simulink model "lab03part1"  (R2015a)
settings: Solver=ode45  StartTime=0.0  StopTime=40.0  RelTol=1e-3
settings Model: Creator=dg  LastModifiedBy=dg

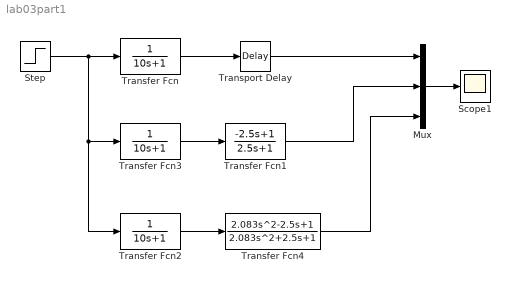
== system lab03part1 ==
  Mux : Mux  Inputs=3
  Scope1 : Scope
  Step : Step  SampleTime=0
  Transfer Fcn : TransferFcn  Denominator=[10 1]
  Transfer Fcn1 : TransferFcn  Numerator=[-2.5 1]  Denominator=[2.5 1]
  Transfer Fcn2 : TransferFcn  Denominator=[10 1]
  Transfer Fcn3 : TransferFcn  Denominator=[10 1]
  Transfer Fcn4 : TransferFcn  Numerator=[2.083 -2.5 1]  Denominator=[2.083 2.5 1]
  Transport Delay : TransportDelay
  wires:
  Step/1 -> Transfer Fcn2/1, Transfer Fcn3/1, Transfer Fcn/1
  Transfer Fcn3/1 -> Transfer Fcn1/1
  Transfer Fcn2/1 -> Transfer Fcn4/1
  Transfer Fcn/1 -> Transport Delay/1
  Transport Delay/1 -> Mux/1
  Transfer Fcn1/1 -> Mux/2
  Transfer Fcn4/1 -> Mux/3
  Mux/1 -> Scope1/1
